simulink model "AcO_Ctrl_Geometric_headless_R2016a"  (R2016a)
settings: Solver=FixedStepDiscrete  StartTime=0.0  StopTime=simulation_duration  FixedStep=Ts  RelTol=1e-3
values from neighbouring files (symbols this model uses):
  M1_BeMo_d = zeros(7,M1_n_mode)    [AcO_Ctrl_headless_cfg.m]    (also in agws_cfg.m = 1e-6*bsxfun(@times,randn(7,M1_n_mode),scale); agws_fastTT_cfg.m = 1e-6*bsxfun(@times,randn(7,M1_n_mode),scale))
  M1_RiBo_d = zeros(7,6)    [AcO_Ctrl_headless_cfg.m]    (also in agws_cfg.m = [M1_Txyz0 M1_Rxyz0]; agws_fastTT_cfg.m = [M1_Txyz0 M1_Rxyz0])
  M2_RiBo_d = zeros(7,6)    [AcO_Ctrl_headless_cfg.m]    (also in agws_cfg.m = [M2_Txyz0 M2_Rxyz0]; agws_fastTT_cfg.m = [M2_Txyz0 M2_Rxyz0])
  Ts = 1/fs    (= 0.002)    [AcO_Ctrl_headless_cfg.m]    (also in agws_fastTT_cfg.m = 0.005)
undefined symbols (not defined in the file or in its folder): Az_C, CG2Hp, CG2Hp_S7, El_C, Fsmm, GIR_C, Hp2CG_f, Hp2CG_f_S7, HPdtf, HpK, KM2, M2_actdyn, M2_CG2Hp, M_LOS, MIMO_C, PTT2act, PTT2act_even, Q, sysd, TT2act, TT2act_even
undefined symbols (not defined in the file): on_axis_src_outputs
libraries: CEO x2
(part 4 of 6)

== system AcO_Ctrl_Geometric_headless_R2016a/Structural Dynamics V3.3/Structural Dynamics V3.5.2/Structural Dynamics Plus CL Az El M1 force/GIR Control ==
  AverageGIRDisp : Inport
  DistributeForces : Gain  Gain=[-ones(2,1);ones(2,1)]  Multiplication=Matrix(K*u)
  GIR Controller : DiscreteFilter  Numerator=GIR_C.num{1}  Denominator=GIR_C.den{1}  SampleTime=1/500
  GIRForces : Outport
  wires:
  AverageGIRDisp/1 -> GIR Controller/1
  DistributeForces/1 -> GIRForces/1
  GIR Controller/1 -> DistributeForces/1

== system AcO_Ctrl_Geometric_headless_R2016a/Structural Dynamics V3.3/Structural Dynamics V3.5.2/Structural Dynamics Plus CL Az El M1 force/M1 Displacement Local Control ==
  note: CG desired displacement/rotation
  note: This block converts from CG displacements and rotations,
      | and converts to Hard Point lengths.  Hard point lengths are
      | changed by applying an equal and opposite force to the hard
      | point, and then offseting output by the commanded change
      | in position.
  note: Hexapod Desired Lengths
  note: Hexapod Offset Forces
  note: Offset displacement, used
      | in calcuation of hard point
      | forces.
  note: The virtual force simulates the extension
      | of the hard point by applying and equal and
      | opposite force on the face of the mirror and cell.
  note: The virtual force simulates the extension
      | of the hard point by applying and equal and
      | opposite force on the face of the mirror and cell.
  M1_cmd(42) : Inport
  CG2Hp{1..6} (6 alike) : Gain  Gain=CG2Hp  Multiplication=Matrix(K*u)
  CG2Hp7 : Gain  Gain=CG2Hp_S7  Multiplication=Matrix(K*u)
  Demux1 : Demux  Outputs=6*ones(7,1)
  Discrete Filter : DiscreteFilter  Numerator=HPdtf.num{1}  Denominator=HPdtf.den{1}
  HpK{1,3..8} (7 alike) : Gain  Gain=HpK  Multiplication=Matrix(K*u)
  Mux1 : Mux  Inputs=6*ones(7,1)
  Mux3 : Mux  Inputs=6*ones(7,1)
  M1_HP_D_cmd(42) : Outport
  M1_HP_F_cmd (42) : Outport  Port=2
  wires:
  HpK3/1 -> Mux3/2
  Mux3/1 -> M1_HP_F_cmd (42)/1
  Mux1/1 -> M1_HP_D_cmd(42)/1
  M1_cmd(42)/1 -> Discrete Filter/1
  Demux1/2 -> CG2Hp1/1
  CG2Hp1/1 -> Mux1/2, HpK3/1
  CG2Hp2/1 -> HpK1/1, Mux1/3
  CG2Hp3/1 -> Mux1/4, HpK4/1
  CG2Hp4/1 -> Mux1/5, HpK5/1
  CG2Hp5/1 -> Mux1/6, HpK6/1
  CG2Hp7/1 -> Mux1/7, HpK7/1
  HpK1/1 -> Mux3/3
  HpK4/1 -> Mux3/4
  HpK5/1 -> Mux3/5
  HpK6/1 -> Mux3/6
  HpK7/1 -> Mux3/7
  Demux1/3 -> CG2Hp2/1
  Demux1/4 -> CG2Hp3/1
  Demux1/5 -> CG2Hp4/1
  Demux1/6 -> CG2Hp5/1
  CG2Hp6/1 -> HpK8/1, Mux1/1
  HpK8/1 -> Mux3/1
  Discrete Filter/1 -> Demux1/1
  Demux1/1 -> CG2Hp6/1
  Demux1/7 -> CG2Hp7/1

== system AcO_Ctrl_Geometric_headless_R2016a/Structural Dynamics V3.3/Structural Dynamics V3.5.2/Structural Dynamics Plus CL Az El M1 force/M1 Force Control ==
  note: in Newtons
  note: Cell Forces (N)
  note: Face Forces (N)
  M1_measured_Force(42) : Inport
  ControlM1S1 : Subsystem
  ControlM1S2 : Subsystem
  ControlM1S3 : Subsystem
  ControlM1S4 : Subsystem
  ControlM1S5 : Subsystem
  ControlM1S6 : Subsystem
  ControlM1S7 : Subsystem
  Demux3 : Demux  Outputs=6*ones(7,1)
  Mux : Mux  Inputs=7
  Mux1 : Mux  Inputs=7
  M1 FaceForce : Outport
  M1 CellForce : Outport  Port=2
  wires:
  M1_measured_Force(42)/1 -> Demux3/1
  Demux3/2 -> ControlM1S2/1(In1)
  Demux3/3 -> ControlM1S3/1(In1)
  Demux3/4 -> ControlM1S4/1(In1)
  Demux3/5 -> ControlM1S5/1(In1)
  Demux3/6 -> ControlM1S6/1(In1)
  ControlM1S1/1(Out1) -> Mux/1
  ControlM1S2/1(Out1) -> Mux/2
  ControlM1S3/1(Out1) -> Mux/3
  ControlM1S4/1(Out1) -> Mux/4
  ControlM1S5/1(Out1) -> Mux/5
  ControlM1S6/1(Out1) -> Mux/6
  ControlM1S7/1(Out1) -> Mux/7
  Mux1/1 -> M1 CellForce/1
  ControlM1S1/2(Out2) -> Mux1/1
  ControlM1S2/2(Out2) -> Mux1/2
  ControlM1S3/2(Out2) -> Mux1/3
  ControlM1S4/2(Out2) -> Mux1/4
  ControlM1S5/2(Out2) -> Mux1/5
  ControlM1S6/2(Out2) -> Mux1/6
  Mux/1 -> M1 FaceForce/1
  Demux3/1 -> ControlM1S1/1(In1)
  ControlM1S7/2(Out2) -> Mux1/7
  Demux3/7 -> ControlM1S7/1(In1)

== system AcO_Ctrl_Geometric_headless_R2016a/Structural Dynamics V3.3/Structural Dynamics V3.5.2/Structural Dynamics Plus CL Az El M1 force/M1 Sensing ==
  M1_cmd (42) : Inport
  M1_HP(84) : Inport  Port=2
  Demux2 : Demux  Outputs=6*ones(14,1)
  Demux9 : Demux  Outputs=6*ones(7,1)
  Mux3 : Mux  Inputs=6*ones(7,1)
  Scope : Scope
  senseM1S1 : Subsystem
  senseM1S2 : Subsystem
  senseM1S3 : Subsystem
  senseM1S4 : Subsystem
  senseM1S5 : Subsystem
  senseM1S6 : Subsystem
  senseM1S7 : Subsystem
  M1 Hard Point Force(42) : Outport
  wires:
  Demux2/9 -> senseM1S5/3(HP_D_cell)
  senseM1S2/1(HardPoint_6DOF_Force) -> Scope/1, Mux3/2
  Demux2/3 -> senseM1S2/3(HP_D_cell)
  Demux2/5 -> senseM1S3/3(HP_D_cell)
  Demux2/7 -> senseM1S4/3(HP_D_cell)
  senseM1S6/1(HardPoint_6DOF_Force) -> Mux3/6
  senseM1S1/1(HardPoint_6DOF_Force) -> Mux3/1
  Demux2/13 -> senseM1S7/3(HP_D_cell)
  Demux2/11 -> senseM1S6/3(HP_D_cell)
  senseM1S5/1(HardPoint_6DOF_Force) -> Mux3/5
  senseM1S4/1(HardPoint_6DOF_Force) -> Mux3/4
  senseM1S3/1(HardPoint_6DOF_Force) -> Mux3/3
  M1_HP(84)/1 -> Demux2/1
  Demux2/1 -> senseM1S1/3(HP_D_cell)
  senseM1S7/1(HardPoint_6DOF_Force) -> Mux3/7
  Mux3/1 -> M1 Hard Point Force(42)/1
  Demux9/2 -> senseM1S2/1(HP_D_cmd)
  Demux9/3 -> senseM1S3/1(HP_D_cmd)
  M1_cmd (42)/1 -> Demux9/1
  Demux9/4 -> senseM1S4/1(HP_D_cmd)
  Demux9/6 -> senseM1S6/1(HP_D_cmd)
  Demux9/1 -> senseM1S1/1(HP_D_cmd)
  Demux9/5 -> senseM1S5/1(HP_D_cmd)
  Demux9/7 -> senseM1S7/1(HP_D_cmd)
  Demux2/2 -> senseM1S1/2(HP_D_face)
  Demux2/4 -> senseM1S2/2(HP_D_face)
  Demux2/6 -> senseM1S3/2(HP_D_face)
  Demux2/8 -> senseM1S4/2(HP_D_face)
  Demux2/10 -> senseM1S5/2(HP_D_face)
  Demux2/12 -> senseM1S6/2(HP_D_face)
  Demux2/14 -> senseM1S7/2(HP_D_face)

== system AcO_Ctrl_Geometric_headless_R2016a/Structural Dynamics V3.3/Structural Dynamics V3.5.2/Structural Dynamics Plus CL Az El M1 force/M2 control ==
  note: M2 actuator Dynamics
  note: Convert from PTT to actuator
      | DOF
  note: in Newtons
  note: in radians
  note: This one is grouped differently so that it is clear that odds and evens are slightly different.
      | Each subsystem controller includes both the TT controller from TT command, to PZT position command, to PZT force (using an open loop approximation).
  note: PTT command (radians)
  note: fancy way of outputting equal and opposite forces
  PTT ref (21) : Inport
  Demux1 : Demux  Outputs=3*ones(7,1)
  M2actuatorDyanmics{1..7} (7 alike) : DiscreteStateSpace  A=M2_actdyn.A  B=M2_actdyn.B  C=M2_actdyn.C  D=M2_actdyn.D  SampleTime=1/Fsmm
  Mux : Mux  Inputs=6*ones(7,1)
  TT_to_act{,1..3} (4 alike) : Gain  Gain=PTT2act  Multiplication=Matrix(K*u)
  TT_to_act4 : Gain  Gain=PTT2act_even  Multiplication=Matrix(K*u)
  TT_to_act5 : Gain  Gain=PTT2act_even  Multiplication=Matrix(K*u)
  TT_to_act6 : Gain  Gain=PTT2act_even  Multiplication=Matrix(K*u)
  delta{1..7} (7 alike) : Gain  Gain=[-eye(3);eye(3)]  Multiplication=Matrix(K*u)
  M2_PZT_F : Outport
  wires:
  M2actuatorDyanmics1/1 -> delta7/1
  TT_to_act/1 -> M2actuatorDyanmics1/1
  M2actuatorDyanmics2/1 -> delta3/1
  TT_to_act1/1 -> M2actuatorDyanmics2/1
  M2actuatorDyanmics3/1 -> delta1/1
  TT_to_act4/1 -> M2actuatorDyanmics3/1
  M2actuatorDyanmics4/1 -> delta2/1
  TT_to_act2/1 -> M2actuatorDyanmics4/1
  M2actuatorDyanmics5/1 -> delta4/1
  TT_to_act5/1 -> M2actuatorDyanmics5/1
  M2actuatorDyanmics6/1 -> delta5/1
  TT_to_act3/1 -> M2actuatorDyanmics6/1
  M2actuatorDyanmics7/1 -> delta6/1
  TT_to_act6/1 -> M2actuatorDyanmics7/1
  PTT ref (21)/1 -> Demux1/1
  Mux/1 -> M2_PZT_F/1
  Demux1/1 -> TT_to_act1/1
  Demux1/2 -> TT_to_act4/1
  Demux1/3 -> TT_to_act2/1
  Demux1/4 -> TT_to_act5/1
  Demux1/5 -> TT_to_act3/1
  Demux1/6 -> TT_to_act6/1
  Demux1/7 -> TT_to_act/1
  delta6/1 -> Mux/6
  delta5/1 -> Mux/5
  delta4/1 -> Mux/4
  delta2/1 -> Mux/3
  delta1/1 -> Mux/2
  delta3/1 -> Mux/1
  delta7/1 -> Mux/7

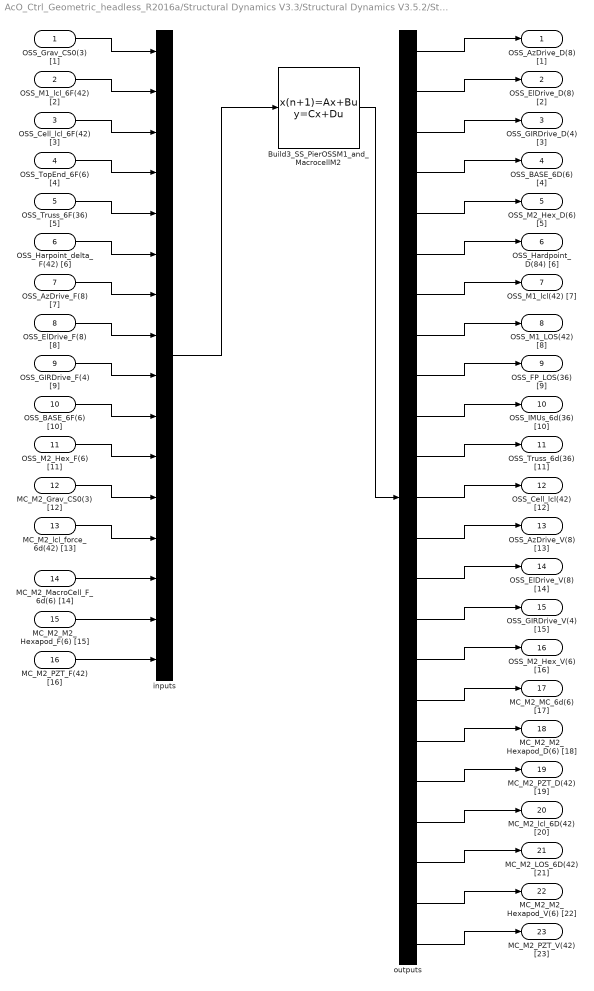
== system AcO_Ctrl_Geometric_headless_R2016a/Structural Dynamics V3.3/Structural Dynamics V3.5.2/Structural Dynamics Plus CL Az El M1 force/PlantDynamics Build3_SS_PierOSSM1_and_MacrocellM2 ==
  OSS_Grav_CS0(3) [1] : Inport  PortDimensions=3
  OSS_M1_lcl_6F(42) [2] : Inport  Port=2  PortDimensions=42
  OSS_Cell_lcl_6F(42) [3] : Inport  Port=3  PortDimensions=42
  OSS_TopEnd_6F(6) [4] : Inport  Port=4  PortDimensions=6
  OSS_Truss_6F(36) [5] : Inport  Port=5  PortDimensions=36
  OSS_Harpoint_delta_F(42) [6] : Inport  Port=6  PortDimensions=42
  OSS_AzDrive_F(8) [7] : Inport  Port=7  PortDimensions=8
  OSS_ElDrive_F(8) [8] : Inport  Port=8  PortDimensions=8
  OSS_GIRDrive_F(4) [9] : Inport  Port=9  PortDimensions=4
  OSS_BASE_6F(6) [10] : Inport  Port=10  PortDimensions=6
  OSS_M2_Hex_F(6) [11] : Inport  Port=11  PortDimensions=6
  MC_M2_Grav_CS0(3) [12] : Inport  Port=12  PortDimensions=3
  MC_M2_lcl_force_6d(42) [13] : Inport  Port=13  PortDimensions=42
  MC_M2_MacroCell_F_6d(6) [14] : Inport  Port=14  PortDimensions=6
  MC_M2_M2_Hexapod_F(6) [15] : Inport  Port=15  PortDimensions=6
  MC_M2_PZT_F(42) [16] : Inport  Port=16  PortDimensions=42
  Build3_SS_PierOSSM1_and_MacrocellM2 : DiscreteStateSpace  A=sysd.sys.A  B=sysd.sys.B  C=sysd.sys.C  D=sysd.sys.D  SampleTime=0.002
  inputs : Mux  Inputs=[3,42,42,6,36,42,8,8,4,6,6,3,42,6,6,42]
  outputs : Demux  Outputs=[8,8,4,6,6,84,42,42,36,36,36,42,8,8,4,6,6,6,42,42,42,6,42]
  OSS_AzDrive_D(8) [1] : Outport  PortDimensions=8
  OSS_ElDrive_D(8) [2] : Outport  Port=2  PortDimensions=8
  OSS_GIRDrive_D(4) [3] : Outport  Port=3  PortDimensions=4
  OSS_BASE_6D(6) [4] : Outport  Port=4  PortDimensions=6
  OSS_M2_Hex_D(6) [5] : Outport  Port=5  PortDimensions=6
  OSS_Hardpoint_D(84) [6] : Outport  Port=6  PortDimensions=84
  OSS_M1_lcl(42) [7] : Outport  Port=7  PortDimensions=42
  OSS_M1_LOS(42) [8] : Outport  Port=8  PortDimensions=42
  OSS_FP_LOS(36) [9] : Outport  Port=9  PortDimensions=36
  OSS_IMUs_6d(36) [10] : Outport  Port=10  PortDimensions=36
  OSS_Truss_6d(36) [11] : Outport  Port=11  PortDimensions=36
  OSS_Cell_lcl(42) [12] : Outport  Port=12  PortDimensions=42
  OSS_AzDrive_V(8) [13] : Outport  Port=13  PortDimensions=8
  OSS_ElDrive_V(8) [14] : Outport  Port=14  PortDimensions=8
  OSS_GIRDrive_V(4) [15] : Outport  Port=15  PortDimensions=4
  OSS_M2_Hex_V(6) [16] : Outport  Port=16  PortDimensions=6
  MC_M2_MC_6d(6) [17] : Outport  Port=17  PortDimensions=6
  MC_M2_M2_Hexapod_D(6) [18] : Outport  Port=18  PortDimensions=6
  MC_M2_PZT_D(42) [19] : Outport  Port=19  PortDimensions=42
  MC_M2_lcl_6D(42) [20] : Outport  Port=20  PortDimensions=42
  MC_M2_LOS_6D(42) [21] : Outport  Port=21  PortDimensions=42
  MC_M2_M2_Hexapod_V(6) [22] : Outport  Port=22  PortDimensions=6
  MC_M2_PZT_V(42) [23] : Outport  Port=23  PortDimensions=42
  wires:
  OSS_Grav_CS0(3) [1]/1 -> inputs/1
  OSS_M1_lcl_6F(42) [2]/1 -> inputs/2
  OSS_Cell_lcl_6F(42) [3]/1 -> inputs/3
  OSS_TopEnd_6F(6) [4]/1 -> inputs/4
  OSS_Truss_6F(36) [5]/1 -> inputs/5
  OSS_Harpoint_delta_F(42) [6]/1 -> inputs/6
  OSS_AzDrive_F(8) [7]/1 -> inputs/7
  OSS_ElDrive_F(8) [8]/1 -> inputs/8
  OSS_GIRDrive_F(4) [9]/1 -> inputs/9
  OSS_BASE_6F(6) [10]/1 -> inputs/10
  OSS_M2_Hex_F(6) [11]/1 -> inputs/11
  MC_M2_Grav_CS0(3) [12]/1 -> inputs/12
  MC_M2_lcl_force_6d(42) [13]/1 -> inputs/13
  MC_M2_MacroCell_F_6d(6) [14]/1 -> inputs/14
  MC_M2_M2_Hexapod_F(6) [15]/1 -> inputs/15
  MC_M2_PZT_F(42) [16]/1 -> inputs/16
  inputs/1 -> Build3_SS_PierOSSM1_and_MacrocellM2/1
  Build3_SS_PierOSSM1_and_MacrocellM2/1 -> outputs/1
  outputs/1 -> OSS_AzDrive_D(8) [1]/1
  outputs/2 -> OSS_ElDrive_D(8) [2]/1
  outputs/3 -> OSS_GIRDrive_D(4) [3]/1
  outputs/4 -> OSS_BASE_6D(6) [4]/1
  outputs/5 -> OSS_M2_Hex_D(6) [5]/1
  outputs/6 -> OSS_Hardpoint_D(84) [6]/1
  outputs/7 -> OSS_M1_lcl(42) [7]/1
  outputs/8 -> OSS_M1_LOS(42) [8]/1
  outputs/9 -> OSS_FP_LOS(36) [9]/1
  outputs/10 -> OSS_IMUs_6d(36) [10]/1
  outputs/11 -> OSS_Truss_6d(36) [11]/1
  outputs/12 -> OSS_Cell_lcl(42) [12]/1
  outputs/13 -> OSS_AzDrive_V(8) [13]/1
  outputs/14 -> OSS_ElDrive_V(8) [14]/1
  outputs/15 -> OSS_GIRDrive_V(4) [15]/1
  outputs/16 -> OSS_M2_Hex_V(6) [16]/1
  outputs/17 -> MC_M2_MC_6d(6) [17]/1
  outputs/18 -> MC_M2_M2_Hexapod_D(6) [18]/1
  outputs/19 -> MC_M2_PZT_D(42) [19]/1
  outputs/20 -> MC_M2_lcl_6D(42) [20]/1
  outputs/21 -> MC_M2_LOS_6D(42) [21]/1
  outputs/22 -> MC_M2_M2_Hexapod_V(6) [22]/1
  outputs/23 -> MC_M2_PZT_V(42) [23]/1

== system AcO_Ctrl_Geometric_headless_R2016a/Structural Dynamics V3.3/Structural Dynamics V3.5.3/Structural Dynamics Plus CL Az El M1 force/Az Control ==
  AverageAzDisp : Inport
  Azimuth Controller : DiscreteFilter  Numerator=Az_C.num{1}  Denominator=Az_C.den{1}  SampleTime=1/500
  DistributeForce : Gain  Gain=[-ones(4,1);ones(4,1)]  Multiplication=Matrix(K*u)
  AzForces : Outport
  wires:
  AverageAzDisp/1 -> Azimuth Controller/1
  DistributeForce/1 -> AzForces/1
  Azimuth Controller/1 -> DistributeForce/1

== system AcO_Ctrl_Geometric_headless_R2016a/Structural Dynamics V3.3/Structural Dynamics V3.5.3/Structural Dynamics Plus CL Az El M1 force/Az El Sensing ==
  note: Note: units are m, not radians for these loops!
      | These loops delta the top and bottom displacements in tangential direction, and average the results.
  Az_disp(8) : Inport
  El_disp(8) : Inport  Port=2
  GIR_disp(4) : Inport  Port=3
  Az : Scope
  Demux : Demux  Outputs=[4,4]
  Demux1 : Demux  Outputs=[4,4]
  Demux2 : Demux  Outputs=[2,2]
  El : Scope
  GIR : Scope
  Sum1 : Sum  Inputs=-+|
  Sum2 : Sum  Inputs=-+|
  Sum3 : Sum  Inputs=-+|
  average : Gain  Gain=ones(1,4)/4  Multiplication=Matrix(K*u)
  average1 : Gain  Gain=ones(1,4)/4  Multiplication=Matrix(K*u)
  average2 : Gain  Gain=ones(1,2)/2  Multiplication=Matrix(K*u)
  El_average(1) : Outport
  Az_average(1) : Outport  Port=2
  GIR_average(1) : Outport  Port=3
  wires:
  average/1 -> El/1, El_average(1)/1
  average1/1 -> Az_average(1)/1, Az/1
  Sum3/1 -> average1/1
  Sum2/1 -> average/1
  Az_disp(8)/1 -> Demux/1
  Demux/2 -> Sum3/2
  Demux/1 -> Sum3/1
  El_disp(8)/1 -> Demux1/1
  Demux1/1 -> Sum2/1
  Demux1/2 -> Sum2/2
  average2/1 -> GIR_average(1)/1, GIR/1
  Sum1/1 -> average2/1
  GIR_disp(4)/1 -> Demux2/1
  Demux2/1 -> Sum1/1
  Demux2/2 -> Sum1/2

== system AcO_Ctrl_Geometric_headless_R2016a/Structural Dynamics V3.3/Structural Dynamics V3.5.3/Structural Dynamics Plus CL Az El M1 force/El Control ==
  AverageElDisp : Inport
  DistributeForces : Gain  Gain=[-ones(4,1);ones(4,1)]  Multiplication=Matrix(K*u)
  Elevation Controller : DiscreteFilter  Numerator=El_C.num{1}  Denominator=El_C.den{1}  SampleTime=1/500
  ElForces : Outport
  wires:
  Elevation Controller/1 -> DistributeForces/1
  DistributeForces/1 -> ElForces/1
  AverageElDisp/1 -> Elevation Controller/1

== system AcO_Ctrl_Geometric_headless_R2016a/Structural Dynamics V3.3/Structural Dynamics V3.5.3/Structural Dynamics Plus CL Az El M1 force/GIR Control ==
  AverageGIRDisp : Inport
  DistributeForces : Gain  Gain=[-ones(2,1);ones(2,1)]  Multiplication=Matrix(K*u)
  GIR Controller : DiscreteFilter  Numerator=GIR_C.num{1}  Denominator=GIR_C.den{1}  SampleTime=1/500
  GIRForces : Outport
  wires:
  AverageGIRDisp/1 -> GIR Controller/1
  DistributeForces/1 -> GIRForces/1
  GIR Controller/1 -> DistributeForces/1

== system AcO_Ctrl_Geometric_headless_R2016a/Structural Dynamics V3.3/Structural Dynamics V3.5.3/Structural Dynamics Plus CL Az El M1 force/M1 Displacement Local Control ==
  note: CG desired displacement/rotation
  note: This block converts from CG displacements and rotations,
      | and converts to Hard Point lengths.  Hard point lengths are
      | changed by applying an equal and opposite force to the hard
      | point, and then offseting output by the commanded change
      | in position.
  note: Hexapod Desired Lengths
  note: Hexapod Offset Forces
  note: Offset displacement, used
      | in calcuation of hard point
      | forces.
  note: The virtual force simulates the extension
      | of the hard point by applying and equal and
      | opposite force on the face of the mirror and cell.
  note: The virtual force simulates the extension
      | of the hard point by applying and equal and
      | opposite force on the face of the mirror and cell.
  M1_cmd(42) : Inport
  CG2Hp{1..6} (6 alike) : Gain  Gain=CG2Hp  Multiplication=Matrix(K*u)
  CG2Hp7 : Gain  Gain=CG2Hp_S7  Multiplication=Matrix(K*u)
  Demux1 : Demux  Outputs=6*ones(7,1)
  Discrete Filter : DiscreteFilter  Numerator=HPdtf.num{1}  Denominator=HPdtf.den{1}
  HpK{1,3..8} (7 alike) : Gain  Gain=HpK  Multiplication=Matrix(K*u)
  Mux1 : Mux  Inputs=6*ones(7,1)
  Mux3 : Mux  Inputs=6*ones(7,1)
  M1_HP_D_cmd(42) : Outport
  M1_HP_F_cmd (42) : Outport  Port=2
  wires:
  HpK3/1 -> Mux3/2
  Mux3/1 -> M1_HP_F_cmd (42)/1
  Mux1/1 -> M1_HP_D_cmd(42)/1
  M1_cmd(42)/1 -> Discrete Filter/1
  Demux1/2 -> CG2Hp1/1
  CG2Hp1/1 -> Mux1/2, HpK3/1
  CG2Hp2/1 -> HpK1/1, Mux1/3
  CG2Hp3/1 -> Mux1/4, HpK4/1
  CG2Hp4/1 -> Mux1/5, HpK5/1
  CG2Hp5/1 -> Mux1/6, HpK6/1
  CG2Hp7/1 -> Mux1/7, HpK7/1
  HpK1/1 -> Mux3/3
  HpK4/1 -> Mux3/4
  HpK5/1 -> Mux3/5
  HpK6/1 -> Mux3/6
  HpK7/1 -> Mux3/7
  Demux1/3 -> CG2Hp2/1
  Demux1/4 -> CG2Hp3/1
  Demux1/5 -> CG2Hp4/1
  Demux1/6 -> CG2Hp5/1
  CG2Hp6/1 -> HpK8/1, Mux1/1
  HpK8/1 -> Mux3/1
  Discrete Filter/1 -> Demux1/1
  Demux1/1 -> CG2Hp6/1
  Demux1/7 -> CG2Hp7/1

== system AcO_Ctrl_Geometric_headless_R2016a/Structural Dynamics V3.3/Structural Dynamics V3.5.3/Structural Dynamics Plus CL Az El M1 force/M1 Force Control ==
  note: in Newtons
  note: Cell Forces (N)
  note: Face Forces (N)
  M1_measured_Force(42) : Inport
  ControlM1S1 : Subsystem
  ControlM1S2 : Subsystem
  ControlM1S3 : Subsystem
  ControlM1S4 : Subsystem
  ControlM1S5 : Subsystem
  ControlM1S6 : Subsystem
  ControlM1S7 : Subsystem
  Demux3 : Demux  Outputs=6*ones(7,1)
  Mux : Mux  Inputs=7
  Mux1 : Mux  Inputs=7
  M1 FaceForce : Outport
  M1 CellForce : Outport  Port=2
  wires:
  M1_measured_Force(42)/1 -> Demux3/1
  Demux3/2 -> ControlM1S2/1(In1)
  Demux3/3 -> ControlM1S3/1(In1)
  Demux3/4 -> ControlM1S4/1(In1)
  Demux3/5 -> ControlM1S5/1(In1)
  Demux3/6 -> ControlM1S6/1(In1)
  ControlM1S1/1(Out1) -> Mux/1
  ControlM1S2/1(Out1) -> Mux/2
  ControlM1S3/1(Out1) -> Mux/3
  ControlM1S4/1(Out1) -> Mux/4
  ControlM1S5/1(Out1) -> Mux/5
  ControlM1S6/1(Out1) -> Mux/6
  ControlM1S7/1(Out1) -> Mux/7
  Mux1/1 -> M1 CellForce/1
  ControlM1S1/2(Out2) -> Mux1/1
  ControlM1S2/2(Out2) -> Mux1/2
  ControlM1S3/2(Out2) -> Mux1/3
  ControlM1S4/2(Out2) -> Mux1/4
  ControlM1S5/2(Out2) -> Mux1/5
  ControlM1S6/2(Out2) -> Mux1/6
  Mux/1 -> M1 FaceForce/1
  Demux3/1 -> ControlM1S1/1(In1)
  ControlM1S7/2(Out2) -> Mux1/7
  Demux3/7 -> ControlM1S7/1(In1)

== system AcO_Ctrl_Geometric_headless_R2016a/Structural Dynamics V3.3/Structural Dynamics V3.5.3/Structural Dynamics Plus CL Az El M1 force/M1 Sensing ==
  M1_cmd (42) : Inport
  M1_HP(84) : Inport  Port=2
  Demux2 : Demux  Outputs=6*ones(14,1)
  Demux9 : Demux  Outputs=6*ones(7,1)
  Mux3 : Mux  Inputs=6*ones(7,1)
  Scope : Scope
  senseM1S1 : Subsystem
  senseM1S2 : Subsystem
  senseM1S3 : Subsystem
  senseM1S4 : Subsystem
  senseM1S5 : Subsystem
  senseM1S6 : Subsystem
  senseM1S7 : Subsystem
  M1 Hard Point Force(42) : Outport
  wires:
  Demux2/9 -> senseM1S5/3(HP_D_cell)
  senseM1S2/1(HardPoint_6DOF_Force) -> Scope/1, Mux3/2
  Demux2/3 -> senseM1S2/3(HP_D_cell)
  Demux2/5 -> senseM1S3/3(HP_D_cell)
  Demux2/7 -> senseM1S4/3(HP_D_cell)
  senseM1S6/1(HardPoint_6DOF_Force) -> Mux3/6
  senseM1S1/1(HardPoint_6DOF_Force) -> Mux3/1
  Demux2/13 -> senseM1S7/3(HP_D_cell)
  Demux2/11 -> senseM1S6/3(HP_D_cell)
  senseM1S5/1(HardPoint_6DOF_Force) -> Mux3/5
  senseM1S4/1(HardPoint_6DOF_Force) -> Mux3/4
  senseM1S3/1(HardPoint_6DOF_Force) -> Mux3/3
  M1_HP(84)/1 -> Demux2/1
  Demux2/1 -> senseM1S1/3(HP_D_cell)
  senseM1S7/1(HardPoint_6DOF_Force) -> Mux3/7
  Mux3/1 -> M1 Hard Point Force(42)/1
  Demux9/2 -> senseM1S2/1(HP_D_cmd)
  Demux9/3 -> senseM1S3/1(HP_D_cmd)
  M1_cmd (42)/1 -> Demux9/1
  Demux9/4 -> senseM1S4/1(HP_D_cmd)
  Demux9/6 -> senseM1S6/1(HP_D_cmd)
  Demux9/1 -> senseM1S1/1(HP_D_cmd)
  Demux9/5 -> senseM1S5/1(HP_D_cmd)
  Demux9/7 -> senseM1S7/1(HP_D_cmd)
  Demux2/2 -> senseM1S1/2(HP_D_face)
  Demux2/4 -> senseM1S2/2(HP_D_face)
  Demux2/6 -> senseM1S3/2(HP_D_face)
  Demux2/8 -> senseM1S4/2(HP_D_face)
  Demux2/10 -> senseM1S5/2(HP_D_face)
  Demux2/12 -> senseM1S6/2(HP_D_face)
  Demux2/14 -> senseM1S7/2(HP_D_face)

== system AcO_Ctrl_Geometric_headless_R2016a/Structural Dynamics V3.3/Structural Dynamics V3.5.3/Structural Dynamics Plus CL Az El M1 force/M2 control ==
  note: M2 actuator Dynamics
  note: Convert from PTT to actuator
      | DOF
  note: in Newtons
  note: in radians
  note: This one is grouped differently so that it is clear that odds and evens are slightly different.
      | Each subsystem controller includes both the TT controller from TT command, to PZT position command, to PZT force (using an open loop approximation).
  note: PTT command (radians)
  note: fancy way of outputting equal and opposite forces
  PTT ref (21) : Inport
  Demux1 : Demux  Outputs=3*ones(7,1)
  M2actuatorDyanmics{1..7} (7 alike) : DiscreteStateSpace  A=M2_actdyn.A  B=M2_actdyn.B  C=M2_actdyn.C  D=M2_actdyn.D  SampleTime=1/Fsmm
  Mux : Mux  Inputs=6*ones(7,1)
  TT_to_act{,1..6} (7 alike) : Gain  Gain=PTT2act  Multiplication=Matrix(K*u)
  delta{1..7} (7 alike) : Gain  Gain=[-eye(3);eye(3)]  Multiplication=Matrix(K*u)
  M2_PZT_F : Outport
  wires:
  M2actuatorDyanmics1/1 -> delta7/1
  TT_to_act/1 -> M2actuatorDyanmics1/1
  M2actuatorDyanmics2/1 -> delta3/1
  TT_to_act1/1 -> M2actuatorDyanmics2/1
  M2actuatorDyanmics3/1 -> delta1/1
  TT_to_act4/1 -> M2actuatorDyanmics3/1
  M2actuatorDyanmics4/1 -> delta2/1
  TT_to_act2/1 -> M2actuatorDyanmics4/1
  M2actuatorDyanmics5/1 -> delta4/1
  TT_to_act5/1 -> M2actuatorDyanmics5/1
  M2actuatorDyanmics6/1 -> delta5/1
  TT_to_act3/1 -> M2actuatorDyanmics6/1
  M2actuatorDyanmics7/1 -> delta6/1
  TT_to_act6/1 -> M2actuatorDyanmics7/1
  PTT ref (21)/1 -> Demux1/1
  Mux/1 -> M2_PZT_F/1
  Demux1/1 -> TT_to_act1/1
  Demux1/2 -> TT_to_act4/1
  Demux1/3 -> TT_to_act2/1
  Demux1/4 -> TT_to_act5/1
  Demux1/5 -> TT_to_act3/1
  Demux1/6 -> TT_to_act6/1
  Demux1/7 -> TT_to_act/1
  delta6/1 -> Mux/6
  delta5/1 -> Mux/5
  delta4/1 -> Mux/4
  delta2/1 -> Mux/3
  delta1/1 -> Mux/2
  delta3/1 -> Mux/1
  delta7/1 -> Mux/7

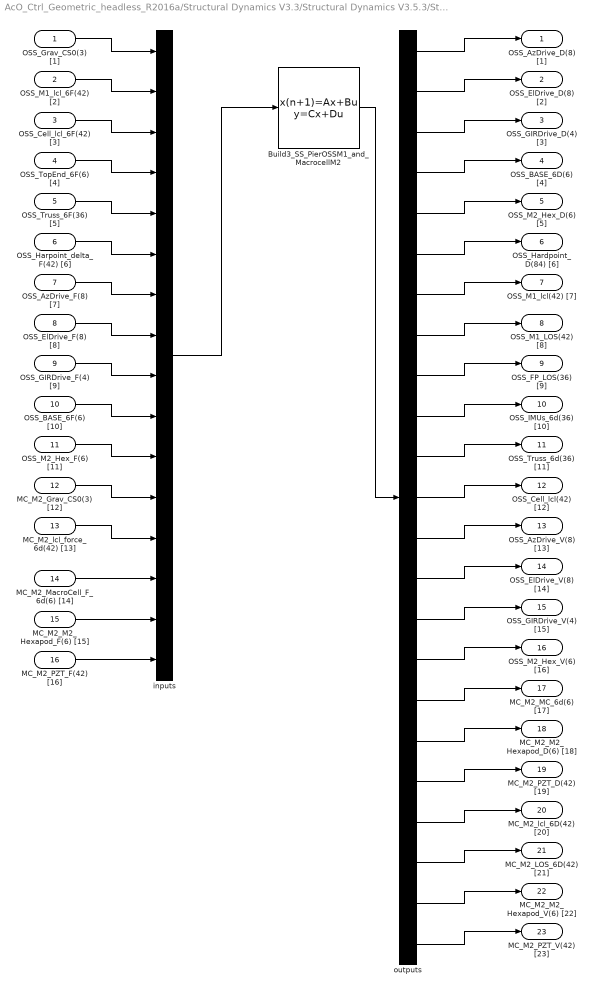
== system AcO_Ctrl_Geometric_headless_R2016a/Structural Dynamics V3.3/Structural Dynamics V3.5.3/Structural Dynamics Plus CL Az El M1 force/PlantDynamics Build3_SS_PierOSSM1_and_MacrocellM2 ==
  OSS_Grav_CS0(3) [1] : Inport  PortDimensions=3
  OSS_M1_lcl_6F(42) [2] : Inport  Port=2  PortDimensions=42
  OSS_Cell_lcl_6F(42) [3] : Inport  Port=3  PortDimensions=42
  OSS_TopEnd_6F(6) [4] : Inport  Port=4  PortDimensions=6
  OSS_Truss_6F(36) [5] : Inport  Port=5  PortDimensions=36
  OSS_Harpoint_delta_F(42) [6] : Inport  Port=6  PortDimensions=42
  OSS_AzDrive_F(8) [7] : Inport  Port=7  PortDimensions=8
  OSS_ElDrive_F(8) [8] : Inport  Port=8  PortDimensions=8
  OSS_GIRDrive_F(4) [9] : Inport  Port=9  PortDimensions=4
  OSS_BASE_6F(6) [10] : Inport  Port=10  PortDimensions=6
  OSS_M2_Hex_F(6) [11] : Inport  Port=11  PortDimensions=6
  MC_M2_Grav_CS0(3) [12] : Inport  Port=12  PortDimensions=3
  MC_M2_lcl_force_6d(42) [13] : Inport  Port=13  PortDimensions=42
  MC_M2_MacroCell_F_6d(6) [14] : Inport  Port=14  PortDimensions=6
  MC_M2_M2_Hexapod_F(6) [15] : Inport  Port=15  PortDimensions=6
  MC_M2_PZT_F(42) [16] : Inport  Port=16  PortDimensions=42
  Build3_SS_PierOSSM1_and_MacrocellM2 : DiscreteStateSpace  A=sysd.sys.A  B=sysd.sys.B  C=sysd.sys.C  D=sysd.sys.D  SampleTime=0.002
  inputs : Mux  Inputs=[3,42,42,6,36,42,8,8,4,6,6,3,42,6,6,42]
  outputs : Demux  Outputs=[8,8,4,6,6,84,42,42,36,36,36,42,8,8,4,6,6,6,42,42,42,6,42]
  OSS_AzDrive_D(8) [1] : Outport  PortDimensions=8
  OSS_ElDrive_D(8) [2] : Outport  Port=2  PortDimensions=8
  OSS_GIRDrive_D(4) [3] : Outport  Port=3  PortDimensions=4
  OSS_BASE_6D(6) [4] : Outport  Port=4  PortDimensions=6
  OSS_M2_Hex_D(6) [5] : Outport  Port=5  PortDimensions=6
  OSS_Hardpoint_D(84) [6] : Outport  Port=6  PortDimensions=84
  OSS_M1_lcl(42) [7] : Outport  Port=7  PortDimensions=42
  OSS_M1_LOS(42) [8] : Outport  Port=8  PortDimensions=42
  OSS_FP_LOS(36) [9] : Outport  Port=9  PortDimensions=36
  OSS_IMUs_6d(36) [10] : Outport  Port=10  PortDimensions=36
  OSS_Truss_6d(36) [11] : Outport  Port=11  PortDimensions=36
  OSS_Cell_lcl(42) [12] : Outport  Port=12  PortDimensions=42
  OSS_AzDrive_V(8) [13] : Outport  Port=13  PortDimensions=8
  OSS_ElDrive_V(8) [14] : Outport  Port=14  PortDimensions=8
  OSS_GIRDrive_V(4) [15] : Outport  Port=15  PortDimensions=4
  OSS_M2_Hex_V(6) [16] : Outport  Port=16  PortDimensions=6
  MC_M2_MC_6d(6) [17] : Outport  Port=17  PortDimensions=6
  MC_M2_M2_Hexapod_D(6) [18] : Outport  Port=18  PortDimensions=6
  MC_M2_PZT_D(42) [19] : Outport  Port=19  PortDimensions=42
  MC_M2_lcl_6D(42) [20] : Outport  Port=20  PortDimensions=42
  MC_M2_LOS_6D(42) [21] : Outport  Port=21  PortDimensions=42
  MC_M2_M2_Hexapod_V(6) [22] : Outport  Port=22  PortDimensions=6
  MC_M2_PZT_V(42) [23] : Outport  Port=23  PortDimensions=42
  wires:
  OSS_Grav_CS0(3) [1]/1 -> inputs/1
  OSS_M1_lcl_6F(42) [2]/1 -> inputs/2
  OSS_Cell_lcl_6F(42) [3]/1 -> inputs/3
  OSS_TopEnd_6F(6) [4]/1 -> inputs/4
  OSS_Truss_6F(36) [5]/1 -> inputs/5
  OSS_Harpoint_delta_F(42) [6]/1 -> inputs/6
  OSS_AzDrive_F(8) [7]/1 -> inputs/7
  OSS_ElDrive_F(8) [8]/1 -> inputs/8
  OSS_GIRDrive_F(4) [9]/1 -> inputs/9
  OSS_BASE_6F(6) [10]/1 -> inputs/10
  OSS_M2_Hex_F(6) [11]/1 -> inputs/11
  MC_M2_Grav_CS0(3) [12]/1 -> inputs/12
  MC_M2_lcl_force_6d(42) [13]/1 -> inputs/13
  MC_M2_MacroCell_F_6d(6) [14]/1 -> inputs/14
  MC_M2_M2_Hexapod_F(6) [15]/1 -> inputs/15
  MC_M2_PZT_F(42) [16]/1 -> inputs/16
  inputs/1 -> Build3_SS_PierOSSM1_and_MacrocellM2/1
  Build3_SS_PierOSSM1_and_MacrocellM2/1 -> outputs/1
  outputs/1 -> OSS_AzDrive_D(8) [1]/1
  outputs/2 -> OSS_ElDrive_D(8) [2]/1
  outputs/3 -> OSS_GIRDrive_D(4) [3]/1
  outputs/4 -> OSS_BASE_6D(6) [4]/1
  outputs/5 -> OSS_M2_Hex_D(6) [5]/1
  outputs/6 -> OSS_Hardpoint_D(84) [6]/1
  outputs/7 -> OSS_M1_lcl(42) [7]/1
  outputs/8 -> OSS_M1_LOS(42) [8]/1
  outputs/9 -> OSS_FP_LOS(36) [9]/1
  outputs/10 -> OSS_IMUs_6d(36) [10]/1
  outputs/11 -> OSS_Truss_6d(36) [11]/1
  outputs/12 -> OSS_Cell_lcl(42) [12]/1
  outputs/13 -> OSS_AzDrive_V(8) [13]/1
  outputs/14 -> OSS_ElDrive_V(8) [14]/1
  outputs/15 -> OSS_GIRDrive_V(4) [15]/1
  outputs/16 -> OSS_M2_Hex_V(6) [16]/1
  outputs/17 -> MC_M2_MC_6d(6) [17]/1
  outputs/18 -> MC_M2_M2_Hexapod_D(6) [18]/1
  outputs/19 -> MC_M2_PZT_D(42) [19]/1
  outputs/20 -> MC_M2_lcl_6D(42) [20]/1
  outputs/21 -> MC_M2_LOS_6D(42) [21]/1
  outputs/22 -> MC_M2_M2_Hexapod_V(6) [22]/1
  outputs/23 -> MC_M2_PZT_V(42) [23]/1

== system AcO_Ctrl_Geometric_headless_R2016a/Structural Dynamics V3.3/Structural Dynamics V3.1/M1 Force Control/ControlM1S1/MIMO Controller ==
  In1 : Inport
  Demux1 : Demux  Outputs=6
  Gain{,1..5} (6 alike) : Gain
  Mux1 : Mux  Inputs=6
  R1 Controller : DiscreteTransferFcn  Numerator=MIMO_C(4,4).num{1}  Denominator=MIMO_C(4,4).den{1}
  R2 Controller : DiscreteTransferFcn  Numerator=MIMO_C(5,5).num{1}  Denominator=MIMO_C(5,5).den{1}
  R3 Controller : DiscreteTransferFcn  Numerator=MIMO_C(6,6).num{1}  Denominator=MIMO_C(6,6).den{1}
  T1 Controller : DiscreteTransferFcn  Numerator=MIMO_C(1,1).num{1}  Denominator=MIMO_C(1,1).den{1}
  T2 Controller : DiscreteTransferFcn  Numerator=MIMO_C(2,2).num{1}  Denominator=MIMO_C(2,2).den{1}
  T3 Controller : DiscreteTransferFcn  Numerator=MIMO_C(3,3).num{1}  Denominator=MIMO_C(3,3).den{1}
  Out1 : Outport
  wires:
  Gain5/1 -> T3 Controller/1
  Gain4/1 -> R3 Controller/1
  Gain3/1 -> R2 Controller/1
  Gain2/1 -> R1 Controller/1
  Gain1/1 -> T2 Controller/1
  Gain/1 -> T1 Controller/1
  Mux1/1 -> Out1/1
  T1 Controller/1 -> Mux1/1
  T2 Controller/1 -> Mux1/2
  T3 Controller/1 -> Mux1/3
  R1 Controller/1 -> Mux1/4
  R2 Controller/1 -> Mux1/5
  R3 Controller/1 -> Mux1/6
  Demux1/6 -> Gain4/1
  Demux1/5 -> Gain3/1
  Demux1/4 -> Gain2/1
  Demux1/3 -> Gain5/1
  Demux1/2 -> Gain1/1
  Demux1/1 -> Gain/1
  In1/1 -> Demux1/1

== system AcO_Ctrl_Geometric_headless_R2016a/Structural Dynamics V3.3/Structural Dynamics V3.1/M1 Force Control/ControlM1S2/MIMO Controller ==
  In1 : Inport
  Demux1 : Demux  Outputs=6
  Gain{,1..5} (6 alike) : Gain
  Mux1 : Mux  Inputs=6
  R1 Controller : DiscreteTransferFcn  Numerator=MIMO_C(4,4).num{1}  Denominator=MIMO_C(4,4).den{1}
  R2 Controller : DiscreteTransferFcn  Numerator=MIMO_C(5,5).num{1}  Denominator=MIMO_C(5,5).den{1}
  R3 Controller : DiscreteTransferFcn  Numerator=MIMO_C(6,6).num{1}  Denominator=MIMO_C(6,6).den{1}
  T1 Controller : DiscreteTransferFcn  Numerator=MIMO_C(1,1).num{1}  Denominator=MIMO_C(1,1).den{1}
  T2 Controller : DiscreteTransferFcn  Numerator=MIMO_C(2,2).num{1}  Denominator=MIMO_C(2,2).den{1}
  T3 Controller : DiscreteTransferFcn  Numerator=MIMO_C(3,3).num{1}  Denominator=MIMO_C(3,3).den{1}
  Out1 : Outport
  wires:
  In1/1 -> Demux1/1
  Demux1/1 -> Gain/1
  Demux1/2 -> Gain1/1
  Demux1/3 -> Gain5/1
  Demux1/4 -> Gain2/1
  Demux1/5 -> Gain3/1
  Demux1/6 -> Gain4/1
  R3 Controller/1 -> Mux1/6
  R2 Controller/1 -> Mux1/5
  R1 Controller/1 -> Mux1/4
  T3 Controller/1 -> Mux1/3
  T2 Controller/1 -> Mux1/2
  T1 Controller/1 -> Mux1/1
  Mux1/1 -> Out1/1
  Gain/1 -> T1 Controller/1
  Gain1/1 -> T2 Controller/1
  Gain2/1 -> R1 Controller/1
  Gain3/1 -> R2 Controller/1
  Gain4/1 -> R3 Controller/1
  Gain5/1 -> T3 Controller/1

== system AcO_Ctrl_Geometric_headless_R2016a/Structural Dynamics V3.3/Structural Dynamics V3.1/M1 Force Control/ControlM1S3/MIMO Controller ==
  In1 : Inport
  Demux1 : Demux  Outputs=6
  Gain{,1..5} (6 alike) : Gain
  Mux1 : Mux  Inputs=6
  R1 Controller : DiscreteTransferFcn  Numerator=MIMO_C(4,4).num{1}  Denominator=MIMO_C(4,4).den{1}
  R2 Controller : DiscreteTransferFcn  Numerator=MIMO_C(5,5).num{1}  Denominator=MIMO_C(5,5).den{1}
  R3 Controller : DiscreteTransferFcn  Numerator=MIMO_C(6,6).num{1}  Denominator=MIMO_C(6,6).den{1}
  T1 Controller : DiscreteTransferFcn  Numerator=MIMO_C(1,1).num{1}  Denominator=MIMO_C(1,1).den{1}
  T2 Controller : DiscreteTransferFcn  Numerator=MIMO_C(2,2).num{1}  Denominator=MIMO_C(2,2).den{1}
  T3 Controller : DiscreteTransferFcn  Numerator=MIMO_C(3,3).num{1}  Denominator=MIMO_C(3,3).den{1}
  Out1 : Outport
  wires:
  Gain5/1 -> T3 Controller/1
  Gain4/1 -> R3 Controller/1
  Gain3/1 -> R2 Controller/1
  Gain2/1 -> R1 Controller/1
  Gain1/1 -> T2 Controller/1
  Gain/1 -> T1 Controller/1
  Mux1/1 -> Out1/1
  T1 Controller/1 -> Mux1/1
  T2 Controller/1 -> Mux1/2
  T3 Controller/1 -> Mux1/3
  R1 Controller/1 -> Mux1/4
  R2 Controller/1 -> Mux1/5
  R3 Controller/1 -> Mux1/6
  Demux1/6 -> Gain4/1
  Demux1/5 -> Gain3/1
  Demux1/4 -> Gain2/1
  Demux1/3 -> Gain5/1
  Demux1/2 -> Gain1/1
  Demux1/1 -> Gain/1
  In1/1 -> Demux1/1

== system AcO_Ctrl_Geometric_headless_R2016a/Structural Dynamics V3.3/Structural Dynamics V3.1/M1 Force Control/ControlM1S4/MIMO Controller ==
  In1 : Inport
  Demux1 : Demux  Outputs=6
  Gain{,1..5} (6 alike) : Gain
  Mux1 : Mux  Inputs=6
  R1 Controller : DiscreteTransferFcn  Numerator=MIMO_C(4,4).num{1}  Denominator=MIMO_C(4,4).den{1}
  R2 Controller : DiscreteTransferFcn  Numerator=MIMO_C(5,5).num{1}  Denominator=MIMO_C(5,5).den{1}
  R3 Controller : DiscreteTransferFcn  Numerator=MIMO_C(6,6).num{1}  Denominator=MIMO_C(6,6).den{1}
  T1 Controller : DiscreteTransferFcn  Numerator=MIMO_C(1,1).num{1}  Denominator=MIMO_C(1,1).den{1}
  T2 Controller : DiscreteTransferFcn  Numerator=MIMO_C(2,2).num{1}  Denominator=MIMO_C(2,2).den{1}
  T3 Controller : DiscreteTransferFcn  Numerator=MIMO_C(3,3).num{1}  Denominator=MIMO_C(3,3).den{1}
  Out1 : Outport
  wires:
  In1/1 -> Demux1/1
  Demux1/1 -> Gain/1
  Demux1/2 -> Gain1/1
  Demux1/3 -> Gain5/1
  Demux1/4 -> Gain2/1
  Demux1/5 -> Gain3/1
  Demux1/6 -> Gain4/1
  R3 Controller/1 -> Mux1/6
  R2 Controller/1 -> Mux1/5
  R1 Controller/1 -> Mux1/4
  T3 Controller/1 -> Mux1/3
  T2 Controller/1 -> Mux1/2
  T1 Controller/1 -> Mux1/1
  Mux1/1 -> Out1/1
  Gain/1 -> T1 Controller/1
  Gain1/1 -> T2 Controller/1
  Gain2/1 -> R1 Controller/1
  Gain3/1 -> R2 Controller/1
  Gain4/1 -> R3 Controller/1
  Gain5/1 -> T3 Controller/1

== system AcO_Ctrl_Geometric_headless_R2016a/Structural Dynamics V3.3/Structural Dynamics V3.1/M1 Force Control/ControlM1S5/MIMO Controller ==
  In1 : Inport
  Demux1 : Demux  Outputs=6
  Gain{,1..5} (6 alike) : Gain
  Mux1 : Mux  Inputs=6
  R1 Controller : DiscreteTransferFcn  Numerator=MIMO_C(4,4).num{1}  Denominator=MIMO_C(4,4).den{1}
  R2 Controller : DiscreteTransferFcn  Numerator=MIMO_C(5,5).num{1}  Denominator=MIMO_C(5,5).den{1}
  R3 Controller : DiscreteTransferFcn  Numerator=MIMO_C(6,6).num{1}  Denominator=MIMO_C(6,6).den{1}
  T1 Controller : DiscreteTransferFcn  Numerator=MIMO_C(1,1).num{1}  Denominator=MIMO_C(1,1).den{1}
  T2 Controller : DiscreteTransferFcn  Numerator=MIMO_C(2,2).num{1}  Denominator=MIMO_C(2,2).den{1}
  T3 Controller : DiscreteTransferFcn  Numerator=MIMO_C(3,3).num{1}  Denominator=MIMO_C(3,3).den{1}
  Out1 : Outport
  wires:
  Gain5/1 -> T3 Controller/1
  Gain4/1 -> R3 Controller/1
  Gain3/1 -> R2 Controller/1
  Gain2/1 -> R1 Controller/1
  Gain1/1 -> T2 Controller/1
  Gain/1 -> T1 Controller/1
  Mux1/1 -> Out1/1
  T1 Controller/1 -> Mux1/1
  T2 Controller/1 -> Mux1/2
  T3 Controller/1 -> Mux1/3
  R1 Controller/1 -> Mux1/4
  R2 Controller/1 -> Mux1/5
  R3 Controller/1 -> Mux1/6
  Demux1/6 -> Gain4/1
  Demux1/5 -> Gain3/1
  Demux1/4 -> Gain2/1
  Demux1/3 -> Gain5/1
  Demux1/2 -> Gain1/1
  Demux1/1 -> Gain/1
  In1/1 -> Demux1/1

== system AcO_Ctrl_Geometric_headless_R2016a/Structural Dynamics V3.3/Structural Dynamics V3.1/M1 Force Control/ControlM1S6/MIMO Controller ==
  In1 : Inport
  Demux1 : Demux  Outputs=6
  Gain{,1..5} (6 alike) : Gain
  Mux1 : Mux  Inputs=6
  R1 Controller : DiscreteTransferFcn  Numerator=MIMO_C(4,4).num{1}  Denominator=MIMO_C(4,4).den{1}
  R2 Controller : DiscreteTransferFcn  Numerator=MIMO_C(5,5).num{1}  Denominator=MIMO_C(5,5).den{1}
  R3 Controller : DiscreteTransferFcn  Numerator=MIMO_C(6,6).num{1}  Denominator=MIMO_C(6,6).den{1}
  T1 Controller : DiscreteTransferFcn  Numerator=MIMO_C(1,1).num{1}  Denominator=MIMO_C(1,1).den{1}
  T2 Controller : DiscreteTransferFcn  Numerator=MIMO_C(2,2).num{1}  Denominator=MIMO_C(2,2).den{1}
  T3 Controller : DiscreteTransferFcn  Numerator=MIMO_C(3,3).num{1}  Denominator=MIMO_C(3,3).den{1}
  Out1 : Outport
  wires:
  In1/1 -> Demux1/1
  Demux1/1 -> Gain/1
  Demux1/2 -> Gain1/1
  Demux1/3 -> Gain5/1
  Demux1/4 -> Gain2/1
  Demux1/5 -> Gain3/1
  Demux1/6 -> Gain4/1
  R3 Controller/1 -> Mux1/6
  R2 Controller/1 -> Mux1/5
  R1 Controller/1 -> Mux1/4
  T3 Controller/1 -> Mux1/3
  T2 Controller/1 -> Mux1/2
  T1 Controller/1 -> Mux1/1
  Mux1/1 -> Out1/1
  Gain/1 -> T1 Controller/1
  Gain1/1 -> T2 Controller/1
  Gain2/1 -> R1 Controller/1
  Gain3/1 -> R2 Controller/1
  Gain4/1 -> R3 Controller/1
  Gain5/1 -> T3 Controller/1

== system AcO_Ctrl_Geometric_headless_R2016a/Structural Dynamics V3.3/Structural Dynamics V3.1/M1 Force Control/ControlM1S7/MIMO Controller ==
  In1 : Inport
  Demux1 : Demux  Outputs=6
  Gain{,1..5} (6 alike) : Gain
  Mux1 : Mux  Inputs=6
  R1 Controller : DiscreteTransferFcn  Numerator=MIMO_C(4,4).num{1}  Denominator=MIMO_C(4,4).den{1}
  R2 Controller : DiscreteTransferFcn  Numerator=MIMO_C(5,5).num{1}  Denominator=MIMO_C(5,5).den{1}
  R3 Controller : DiscreteTransferFcn  Numerator=MIMO_C(6,6).num{1}  Denominator=MIMO_C(6,6).den{1}
  T1 Controller : DiscreteTransferFcn  Numerator=MIMO_C(1,1).num{1}  Denominator=MIMO_C(1,1).den{1}
  T2 Controller : DiscreteTransferFcn  Numerator=MIMO_C(2,2).num{1}  Denominator=MIMO_C(2,2).den{1}
  T3 Controller : DiscreteTransferFcn  Numerator=MIMO_C(3,3).num{1}  Denominator=MIMO_C(3,3).den{1}
  Out1 : Outport
  wires:
  Gain5/1 -> T3 Controller/1
  Gain4/1 -> R3 Controller/1
  Gain3/1 -> R2 Controller/1
  Gain2/1 -> R1 Controller/1
  Gain1/1 -> T2 Controller/1
  Gain/1 -> T1 Controller/1
  Mux1/1 -> Out1/1
  T1 Controller/1 -> Mux1/1
  T2 Controller/1 -> Mux1/2
  T3 Controller/1 -> Mux1/3
  R1 Controller/1 -> Mux1/4
  R2 Controller/1 -> Mux1/5
  R3 Controller/1 -> Mux1/6
  Demux1/6 -> Gain4/1
  Demux1/5 -> Gain3/1
  Demux1/4 -> Gain2/1
  Demux1/3 -> Gain5/1
  Demux1/2 -> Gain1/1
  Demux1/1 -> Gain/1
  In1/1 -> Demux1/1

== system AcO_Ctrl_Geometric_headless_R2016a/Structural Dynamics V3.3/Structural Dynamics V3.3/Structural Dynamics Plus CL Az El M1 force/M1 Force Control/ControlM1S1 ==
  In1 : Inport
  -1(2)3 : Gain  Gain=-1
  Actuator Model : DiscreteStateSpace  A=Q.A  B=Q.B  C=Q.C  D=Q.D  SampleTime=1/Fsmm
  MIMO Controller : Subsystem
  Out1 : Outport
  Out2 : Outport  Port=2
  wires:
  MIMO Controller/1(Out1) -> Actuator Model/1
  -1(2)3/1 -> Out2/1
  Actuator Model/1 -> -1(2)3/1, Out1/1
  In1/1 -> MIMO Controller/1(In1)

== system AcO_Ctrl_Geometric_headless_R2016a/Structural Dynamics V3.3/Structural Dynamics V3.3/Structural Dynamics Plus CL Az El M1 force/M1 Force Control/ControlM1S2 ==
  In1 : Inport
  -1(2)3 : Gain  Gain=-1
  Actuator Model : DiscreteStateSpace  A=Q.A  B=Q.B  C=Q.C  D=Q.D  SampleTime=1/Fsmm
  MIMO Controller : Subsystem
  Out1 : Outport
  Out2 : Outport  Port=2
  wires:
  In1/1 -> MIMO Controller/1(In1)
  Actuator Model/1 -> Out1/1, -1(2)3/1
  -1(2)3/1 -> Out2/1
  MIMO Controller/1(Out1) -> Actuator Model/1

== system AcO_Ctrl_Geometric_headless_R2016a/Structural Dynamics V3.3/Structural Dynamics V3.3/Structural Dynamics Plus CL Az El M1 force/M1 Force Control/ControlM1S3 ==
  In1 : Inport
  -1(2)3 : Gain  Gain=-1
  Actuator Model : DiscreteStateSpace  A=Q.A  B=Q.B  C=Q.C  D=Q.D  SampleTime=1/Fsmm
  MIMO Controller : Subsystem
  Out1 : Outport
  Out2 : Outport  Port=2
  wires:
  MIMO Controller/1(Out1) -> Actuator Model/1
  -1(2)3/1 -> Out2/1
  Actuator Model/1 -> -1(2)3/1, Out1/1
  In1/1 -> MIMO Controller/1(In1)

== system AcO_Ctrl_Geometric_headless_R2016a/Structural Dynamics V3.3/Structural Dynamics V3.3/Structural Dynamics Plus CL Az El M1 force/M1 Force Control/ControlM1S4 ==
  In1 : Inport
  -1(2)3 : Gain  Gain=-1
  Actuator Model : DiscreteStateSpace  A=Q.A  B=Q.B  C=Q.C  D=Q.D  SampleTime=1/Fsmm
  MIMO Controller : Subsystem
  Out1 : Outport
  Out2 : Outport  Port=2
  wires:
  In1/1 -> MIMO Controller/1(In1)
  Actuator Model/1 -> Out1/1, -1(2)3/1
  -1(2)3/1 -> Out2/1
  MIMO Controller/1(Out1) -> Actuator Model/1

== system AcO_Ctrl_Geometric_headless_R2016a/Structural Dynamics V3.3/Structural Dynamics V3.3/Structural Dynamics Plus CL Az El M1 force/M1 Force Control/ControlM1S5 ==
  In1 : Inport
  -1(2)3 : Gain  Gain=-1
  Actuator Model : DiscreteStateSpace  A=Q.A  B=Q.B  C=Q.C  D=Q.D  SampleTime=1/Fsmm
  MIMO Controller : Subsystem
  Out1 : Outport
  Out2 : Outport  Port=2
  wires:
  MIMO Controller/1(Out1) -> Actuator Model/1
  -1(2)3/1 -> Out2/1
  Actuator Model/1 -> -1(2)3/1, Out1/1
  In1/1 -> MIMO Controller/1(In1)

== system AcO_Ctrl_Geometric_headless_R2016a/Structural Dynamics V3.3/Structural Dynamics V3.3/Structural Dynamics Plus CL Az El M1 force/M1 Force Control/ControlM1S6 ==
  In1 : Inport
  -1(2)3 : Gain  Gain=-1
  Actuator Model : DiscreteStateSpace  A=Q.A  B=Q.B  C=Q.C  D=Q.D  SampleTime=1/Fsmm
  MIMO Controller : Subsystem
  Out1 : Outport
  Out2 : Outport  Port=2
  wires:
  In1/1 -> MIMO Controller/1(In1)
  Actuator Model/1 -> Out1/1, -1(2)3/1
  -1(2)3/1 -> Out2/1
  MIMO Controller/1(Out1) -> Actuator Model/1

== system AcO_Ctrl_Geometric_headless_R2016a/Structural Dynamics V3.3/Structural Dynamics V3.3/Structural Dynamics Plus CL Az El M1 force/M1 Force Control/ControlM1S7 ==
  In1 : Inport
  -1(2)3 : Gain  Gain=-1
  Actuator Model : DiscreteStateSpace  A=Q.A  B=Q.B  C=Q.C  D=Q.D  SampleTime=1/Fsmm
  MIMO Controller : Subsystem
  Out1 : Outport
  Out2 : Outport  Port=2
  wires:
  In1/1 -> MIMO Controller/1(In1)
  Actuator Model/1 -> Out1/1, -1(2)3/1
  -1(2)3/1 -> Out2/1
  MIMO Controller/1(Out1) -> Actuator Model/1

== system AcO_Ctrl_Geometric_headless_R2016a/Structural Dynamics V3.3/Structural Dynamics V3.3/Structural Dynamics Plus CL Az El M1 force/M1 Sensing/senseM1S1 ==
  HP_D_cmd : Inport
  HP_D_face : Inport  Port=2
  HP_D_cell : Inport  Port=3
  Hp2CG_f : Gain  Gain=Hp2CG_f  Multiplication=Matrix(K*u)
  KHp : Gain  Gain=-HpK
  Scope : Scope
  Sum1 : Sum  Inputs=-+|
  Sum9 : Sum  Inputs=-+|
  HardPoint_6DOF_Force : Outport
  wires:
  HP_D_cell/1 -> Sum9/1
  Sum1/1 -> KHp/1
  Hp2CG_f/1 -> HardPoint_6DOF_Force/1
  KHp/1 -> Hp2CG_f/1
  Sum9/1 -> Sum1/2, Scope/1
  HP_D_cmd/1 -> Sum1/1
  HP_D_face/1 -> Sum9/2

== system AcO_Ctrl_Geometric_headless_R2016a/Structural Dynamics V3.3/Structural Dynamics V3.3/Structural Dynamics Plus CL Az El M1 force/M1 Sensing/senseM1S2 ==
  HP_D_cmd : Inport
  HP_D_face : Inport  Port=2
  HP_D_cell : Inport  Port=3
  Hp2CG_f : Gain  Gain=Hp2CG_f  Multiplication=Matrix(K*u)
  KHp : Gain  Gain=-HpK
  Sum1 : Sum  Inputs=-+|
  Sum9 : Sum  Inputs=-+|
  HardPoint_6DOF_Force : Outport
  wires:
  KHp/1 -> Hp2CG_f/1
  Sum1/1 -> KHp/1
  Sum9/1 -> Sum1/2
  Hp2CG_f/1 -> HardPoint_6DOF_Force/1
  HP_D_cell/1 -> Sum9/1
  HP_D_cmd/1 -> Sum1/1
  HP_D_face/1 -> Sum9/2

== system AcO_Ctrl_Geometric_headless_R2016a/Structural Dynamics V3.3/Structural Dynamics V3.3/Structural Dynamics Plus CL Az El M1 force/M1 Sensing/senseM1S3 ==
  HP_D_cmd : Inport
  HP_D_face : Inport  Port=2
  HP_D_cell : Inport  Port=3
  Hp2CG_f : Gain  Gain=Hp2CG_f  Multiplication=Matrix(K*u)
  KHp : Gain  Gain=-HpK
  Sum1 : Sum  Inputs=-+|
  Sum9 : Sum  Inputs=-+|
  HardPoint_6DOF_Force : Outport
  wires:
  KHp/1 -> Hp2CG_f/1
  Sum1/1 -> KHp/1
  Sum9/1 -> Sum1/2
  HP_D_face/1 -> Sum9/2
  HP_D_cmd/1 -> Sum1/1
  HP_D_cell/1 -> Sum9/1
  Hp2CG_f/1 -> HardPoint_6DOF_Force/1

== system AcO_Ctrl_Geometric_headless_R2016a/Structural Dynamics V3.3/Structural Dynamics V3.3/Structural Dynamics Plus CL Az El M1 force/M1 Sensing/senseM1S4 ==
  HP_D_cmd : Inport
  HP_D_face : Inport  Port=2
  HP_D_cell : Inport  Port=3
  Hp2CG_f : Gain  Gain=Hp2CG_f  Multiplication=Matrix(K*u)
  KHp : Gain  Gain=-HpK
  Sum1 : Sum  Inputs=-+|
  Sum9 : Sum  Inputs=-+|
  HardPoint_6DOF_Force : Outport
  wires:
  KHp/1 -> Hp2CG_f/1
  Sum1/1 -> KHp/1
  Sum9/1 -> Sum1/2
  Hp2CG_f/1 -> HardPoint_6DOF_Force/1
  HP_D_cell/1 -> Sum9/1
  HP_D_cmd/1 -> Sum1/1
  HP_D_face/1 -> Sum9/2

== system AcO_Ctrl_Geometric_headless_R2016a/Structural Dynamics V3.3/Structural Dynamics V3.3/Structural Dynamics Plus CL Az El M1 force/M1 Sensing/senseM1S5 ==
  HP_D_cmd : Inport
  HP_D_face : Inport  Port=2
  HP_D_cell : Inport  Port=3
  Hp2CG_f : Gain  Gain=Hp2CG_f  Multiplication=Matrix(K*u)
  KHp : Gain  Gain=-HpK
  Sum1 : Sum  Inputs=-+|
  Sum9 : Sum  Inputs=-+|
  HardPoint_6DOF_Force : Outport
  wires:
  KHp/1 -> Hp2CG_f/1
  Sum1/1 -> KHp/1
  Sum9/1 -> Sum1/2
  HP_D_face/1 -> Sum9/2
  HP_D_cmd/1 -> Sum1/1
  HP_D_cell/1 -> Sum9/1
  Hp2CG_f/1 -> HardPoint_6DOF_Force/1

== system AcO_Ctrl_Geometric_headless_R2016a/Structural Dynamics V3.3/Structural Dynamics V3.3/Structural Dynamics Plus CL Az El M1 force/M1 Sensing/senseM1S6 ==
  HP_D_cmd : Inport
  HP_D_face : Inport  Port=2
  HP_D_cell : Inport  Port=3
  Hp2CG_f : Gain  Gain=Hp2CG_f  Multiplication=Matrix(K*u)
  KHp : Gain  Gain=-HpK
  Sum1 : Sum  Inputs=-+|
  Sum9 : Sum  Inputs=-+|
  HardPoint_6DOF_Force : Outport
  wires:
  KHp/1 -> Hp2CG_f/1
  Sum1/1 -> KHp/1
  Sum9/1 -> Sum1/2
  Hp2CG_f/1 -> HardPoint_6DOF_Force/1
  HP_D_cell/1 -> Sum9/1
  HP_D_cmd/1 -> Sum1/1
  HP_D_face/1 -> Sum9/2

== system AcO_Ctrl_Geometric_headless_R2016a/Structural Dynamics V3.3/Structural Dynamics V3.3/Structural Dynamics Plus CL Az El M1 force/M1 Sensing/senseM1S7 ==
  HP_D_cmd : Inport
  HP_D_face : Inport  Port=2
  HP_D_cell : Inport  Port=3
  Hp2CG_f_S7 : Gain  Gain=Hp2CG_f_S7  Multiplication=Matrix(K*u)
  KHp : Gain  Gain=-HpK
  Sum1 : Sum  Inputs=-+|
  Sum9 : Sum  Inputs=-+|
  HardPoint_6DOF_Force : Outport
  wires:
  KHp/1 -> Hp2CG_f_S7/1
  Sum1/1 -> KHp/1
  Sum9/1 -> Sum1/2
  HP_D_face/1 -> Sum9/2
  HP_D_cmd/1 -> Sum1/1
  HP_D_cell/1 -> Sum9/1
  Hp2CG_f_S7/1 -> HardPoint_6DOF_Force/1

== system AcO_Ctrl_Geometric_headless_R2016a/Structural Dynamics V3.3/Structural Dynamics V3.3a/Structural Dynamics Plus CL Az El M1 force/M1 Force Control/ControlM1S1 ==
  In1 : Inport
  -1(2)3 : Gain  Gain=-1
  Actuator Model : DiscreteStateSpace  A=Q.A  B=Q.B  C=Q.C  D=Q.D  SampleTime=1/Fsmm
  MIMO Controller : Subsystem
  Out1 : Outport
  Out2 : Outport  Port=2
  wires:
  In1/1 -> MIMO Controller/1(In1)
  Actuator Model/1 -> Out1/1, -1(2)3/1
  -1(2)3/1 -> Out2/1
  MIMO Controller/1(Out1) -> Actuator Model/1

== system AcO_Ctrl_Geometric_headless_R2016a/Structural Dynamics V3.3/Structural Dynamics V3.3a/Structural Dynamics Plus CL Az El M1 force/M1 Force Control/ControlM1S2 ==
  In1 : Inport
  -1(2)3 : Gain  Gain=-1
  Actuator Model : DiscreteStateSpace  A=Q.A  B=Q.B  C=Q.C  D=Q.D  SampleTime=1/Fsmm
  MIMO Controller : Subsystem
  Out1 : Outport
  Out2 : Outport  Port=2
  wires:
  MIMO Controller/1(Out1) -> Actuator Model/1
  -1(2)3/1 -> Out2/1
  Actuator Model/1 -> -1(2)3/1, Out1/1
  In1/1 -> MIMO Controller/1(In1)

== system AcO_Ctrl_Geometric_headless_R2016a/Structural Dynamics V3.3/Structural Dynamics V3.3a/Structural Dynamics Plus CL Az El M1 force/M1 Force Control/ControlM1S3 ==
  In1 : Inport
  -1(2)3 : Gain  Gain=-1
  Actuator Model : DiscreteStateSpace  A=Q.A  B=Q.B  C=Q.C  D=Q.D  SampleTime=1/Fsmm
  MIMO Controller : Subsystem
  Out1 : Outport
  Out2 : Outport  Port=2
  wires:
  In1/1 -> MIMO Controller/1(In1)
  Actuator Model/1 -> Out1/1, -1(2)3/1
  -1(2)3/1 -> Out2/1
  MIMO Controller/1(Out1) -> Actuator Model/1

== system AcO_Ctrl_Geometric_headless_R2016a/Structural Dynamics V3.3/Structural Dynamics V3.3a/Structural Dynamics Plus CL Az El M1 force/M1 Force Control/ControlM1S4 ==
  In1 : Inport
  -1(2)3 : Gain  Gain=-1
  Actuator Model : DiscreteStateSpace  A=Q.A  B=Q.B  C=Q.C  D=Q.D  SampleTime=1/Fsmm
  MIMO Controller : Subsystem
  Out1 : Outport
  Out2 : Outport  Port=2
  wires:
  MIMO Controller/1(Out1) -> Actuator Model/1
  -1(2)3/1 -> Out2/1
  Actuator Model/1 -> -1(2)3/1, Out1/1
  In1/1 -> MIMO Controller/1(In1)

== system AcO_Ctrl_Geometric_headless_R2016a/Structural Dynamics V3.3/Structural Dynamics V3.3a/Structural Dynamics Plus CL Az El M1 force/M1 Force Control/ControlM1S5 ==
  In1 : Inport
  -1(2)3 : Gain  Gain=-1
  Actuator Model : DiscreteStateSpace  A=Q.A  B=Q.B  C=Q.C  D=Q.D  SampleTime=1/Fsmm
  MIMO Controller : Subsystem
  Out1 : Outport
  Out2 : Outport  Port=2
  wires:
  In1/1 -> MIMO Controller/1(In1)
  Actuator Model/1 -> Out1/1, -1(2)3/1
  -1(2)3/1 -> Out2/1
  MIMO Controller/1(Out1) -> Actuator Model/1

== system AcO_Ctrl_Geometric_headless_R2016a/Structural Dynamics V3.3/Structural Dynamics V3.3a/Structural Dynamics Plus CL Az El M1 force/M1 Force Control/ControlM1S6 ==
  In1 : Inport
  -1(2)3 : Gain  Gain=-1
  Actuator Model : DiscreteStateSpace  A=Q.A  B=Q.B  C=Q.C  D=Q.D  SampleTime=1/Fsmm
  MIMO Controller : Subsystem
  Out1 : Outport
  Out2 : Outport  Port=2
  wires:
  MIMO Controller/1(Out1) -> Actuator Model/1
  -1(2)3/1 -> Out2/1
  Actuator Model/1 -> -1(2)3/1, Out1/1
  In1/1 -> MIMO Controller/1(In1)

== system AcO_Ctrl_Geometric_headless_R2016a/Structural Dynamics V3.3/Structural Dynamics V3.3a/Structural Dynamics Plus CL Az El M1 force/M1 Force Control/ControlM1S7 ==
  In1 : Inport
  -1(2)3 : Gain  Gain=-1
  Actuator Model : DiscreteStateSpace  A=Q.A  B=Q.B  C=Q.C  D=Q.D  SampleTime=1/Fsmm
  MIMO Controller : Subsystem
  Out1 : Outport
  Out2 : Outport  Port=2
  wires:
  MIMO Controller/1(Out1) -> Actuator Model/1
  -1(2)3/1 -> Out2/1
  Actuator Model/1 -> -1(2)3/1, Out1/1
  In1/1 -> MIMO Controller/1(In1)

== system AcO_Ctrl_Geometric_headless_R2016a/Structural Dynamics V3.3/Structural Dynamics V3.3a/Structural Dynamics Plus CL Az El M1 force/M1 Sensing/senseM1S1 ==
  HP_D_cmd : Inport
  HP_D_face : Inport  Port=2
  HP_D_cell : Inport  Port=3
  Hp2CG_f : Gain  Gain=Hp2CG_f  Multiplication=Matrix(K*u)
  KHp : Gain  Gain=-HpK
  Scope : Scope
  Sum1 : Sum  Inputs=-+|
  Sum9 : Sum  Inputs=-+|
  HardPoint_6DOF_Force : Outport
  wires:
  HP_D_face/1 -> Sum9/2
  HP_D_cmd/1 -> Sum1/1
  Sum9/1 -> Scope/1, Sum1/2
  KHp/1 -> Hp2CG_f/1
  Hp2CG_f/1 -> HardPoint_6DOF_Force/1
  Sum1/1 -> KHp/1
  HP_D_cell/1 -> Sum9/1
